simulink model "proba_model"  (R2016a)
settings: Solver=VariableStepAuto  StartTime=0.0  StopTime=1000  RelTol=1e-3
undefined symbols (not defined in the file or in its folder): sigbuilder_block
settings Model: Creator=user  LastModifiedBy=user

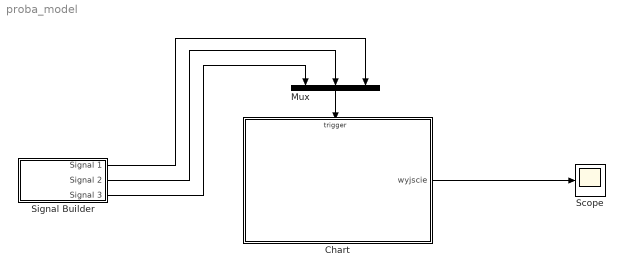
== system proba_model ==
  Chart : Stateflow chart  TreatAsAtomicUnit=on
  Mux : Mux  Inputs=3
  Scope : Scope
  Signal Builder : Subsystem  Tag=STV Subsys  LoadFcn=sigbuilder_block('load');  StartFcn=sigbuilder_block('start');  StopFcn=sigbuilder_block('stop');  ClipboardFcn=sigbuilder_block('clipboard');  mask(Sigbuilder block){}
      mask help: Simulink:masks:SigbuilderBlock_MD
      mask init:
      | if ~strcmp(get_param(bdroot(gcbh),'SimulationStatus'),'stopped') tuvar = sigbuilder_block('maskInit'); end
      settings: CopyFcn=sigbuilder_block('copy');  DeleteFcn=sigbuilder_block('delete');  ModelCloseFcn=sigbuilder_block('modelClose');  PreSaveFcn=sigbuilder_block('preSave');  PauseFcn=sigbuilder_block('pause');  ContinueFcn=sigbuilder_block('continue');  NameChangeFcn=sigbuilder_block('namechange');  OpenFcn=sigbuilder_block('open',[437.6 199.2 550.4 400 ]);  CloseFcn=sigbuilder_block('close');
      mask Display: plot(0, 0, 100, 100,[2, 2, 32, 32, 2], [68, 8, 8, 68, 68],[32, 2], [38, 38], [32, 19, 2],[53, 60, 44], [32, 17, 17, 2],[16, 16, 31, 31]);txt = getActiveGroup(gcbh);text(2, 100, txt,'verticalAlignment', 'top');
  wires:
  Mux/1 -> Chart/Trigger
  Signal Builder/1(Signal 1) -> Mux/3
  Signal Builder/2(Signal 2) -> Mux/2
  Signal Builder/3(Signal 3) -> Mux/1
  Chart/1(wyjscie) -> Scope/1

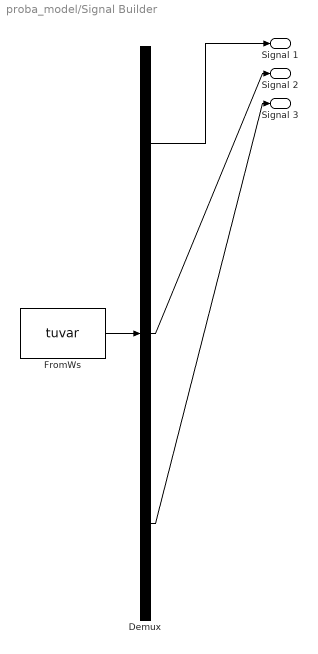
== system proba_model/Signal Builder ==
  Demux : Demux  Tag=STV Demux  Outputs=3
  FromWs : FromWorkspace  Tag=STV FromWs  VariableName=tuvar  SampleTime=0
      SigBuilderData=|
      | common.afterFinalStr = 'Extrapolate'
      | common.sampleTime = 0
      | dataSet.timeRange = [0 10]
      | dataSet.name = 'Group 1'
      | sbobj.Groups.Name = 'Group 1'
      | sbobj.Groups.Signals(1).Name = 'Signal 1'
      | sbobj.Groups.Signals(1).XData = [0 7 7 8 8 10]
      | sbobj.Groups.Signals(1).YData = [0 0 1 1 0 0]
      | sbobj.Groups.Signals(2).Name = 'Signal 2'
      | sbobj.Groups.Signals(2).XData = [0 0.98 0.98 1.98 1.98 10]
      | sbobj.Groups.Signals(2).YData = [0 0 1 1 0 0]
      | sbobj.Groups.Signals(3).Name = 'Signal 3'
      | sbobj.Groups.Signals(3).XData = [0 3 3 3.98 3.98 10]
      | sbobj.Groups.Signals(3).YData = [0 0 1 1 0 0]
  Signal 1 : Outport  Tag=STV Outport
  Signal 2 : Outport  Tag=STV Outport  Port=2
  Signal 3 : Outport  Tag=STV Outport  Port=3
  wires:
  Demux/1 -> Signal 1/1
  FromWs/1 -> Demux/1
  Demux/2 -> Signal 2/1
  Demux/3 -> Signal 3/1

== stateflow chart proba_model/Chart ==
  state stop
    du: wyjscie=0;
  state stan_down
    en:
    level=level-1;
    down=down-1;
    du: wyjscie=-1;
    on Signal_1: down=down+1;
  state stan_up
    en:
    level=level+1;
    up=up-1;
    du: wyjscie=1;
    on Signal_3: up=up+1;
  (default) -> stop
  stop -> stan_down [order 1] : after(30,secs)
  stop -> stan_down [order 7] : Signal_1[level==3]{down=2}
  stop -> stan_up [order 4] : Signal_3[level==1]{up=2}
  stop -> stan_up [order 3] : Signal_3[level==2]{up=1}
  stop -> stan_up [order 2] : Signal_2[level==1]{up=1}
  stop -> stan_down [order 6] : Signal_1[level==2]{down=1}
  stop -> stan_down [order 5] : Signal_2[level==3]{down=1}
  stan_up -> stop [order 2] : [level==3]
  stan_up -> stop [order 3] : [up==0]
  stan_down -> stop [order 3] : [down==0]
  stan_down -> stop [order 2] : [level==1]
  stan_down -> stan_down [order 1] : [down==1]
  stan_up -> stan_up [order 1] : [up==1]
  data: wyjscie output double =0; up local double =0; level local double =1; down local double =0
  events: Signal_1 input RISING_EDGE_EVENT; Signal_2 input RISING_EDGE_EVENT; Signal_3 input RISING_EDGE_EVENT; secs local FUNCTION_CALL_EVENT
